simulink model "Week1_problem3"  (R2020b)
settings: Solver=VariableStepAuto  StartTime=0.0  StopTime=10.0  RelTol=1e-3
settings Model: Creator=gauri  LastModifiedBy=mluser

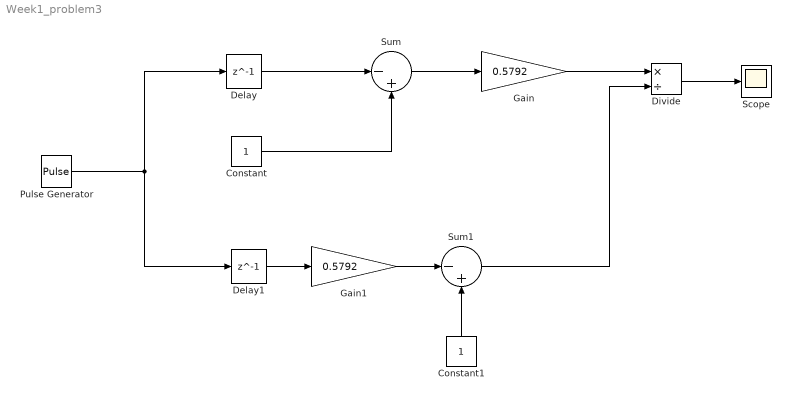
== system Week1_problem3 ==
  Constant : Constant
  Constant1 : Constant
  Delay : Delay  DelayLength=1  InitialCondition=0
  Delay1 : Delay  DelayLength=1  InitialCondition=0
  Divide : Product  Inputs=*/
  Gain : Gain  Gain=0.5792
  Gain1 : Gain  Gain=0.5792
  Pulse Generator : DiscretePulseGenerator  PulseType=Time based  Period=10  PulseWidth=5
  Scope : Scope
  Sum : Sum  Inputs=|-+
  Sum1 : Sum  Inputs=|-+
  wires:
  Delay/1 -> Sum/1
  Constant/1 -> Sum/2
  Pulse Generator/1 -> Delay/1, Delay1/1
  Sum/1 -> Gain/1
  Delay1/1 -> Gain1/1
  Gain1/1 -> Sum1/1
  Constant1/1 -> Sum1/2
  Gain/1 -> Divide/1
  Sum1/1 -> Divide/2
  Divide/1 -> Scope/1
